simulink library "SUB_L4_Task_20ms"  (R2018a)
settings: Solver=VariableStepAuto  StartTime=0.0  StopTime=10.0  RelTol=1e-3
undefined symbols (not defined in the file or in its folder): DiscIntNeverNeededParam
settings Model: Creator=Chris.Balton  LastModifiedBy=Chris.Balton

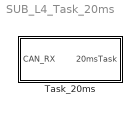
== system SUB_L4_Task_20ms ==
  Task_20ms : Subsystem  TreatAsAtomicUnit=on  SystemSampleTime=0.02

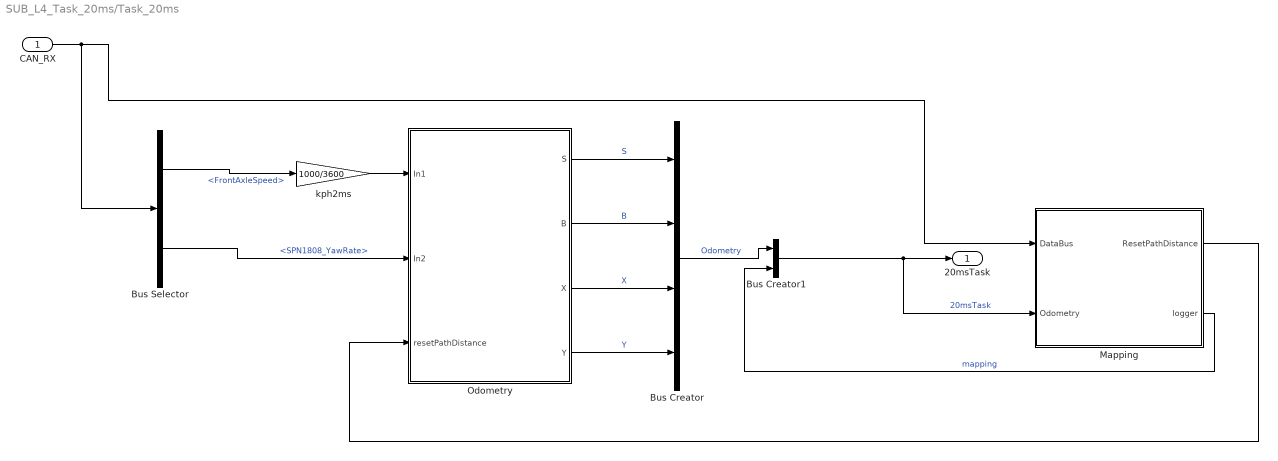
== system SUB_L4_Task_20ms/Task_20ms ==
  CAN_RX : Inport
  Bus Creator : BusCreator  Inputs=4
  Bus Creator1 : BusCreator  Inputs=2
  Bus Selector : BusSelector  OutputSignals=CAN.EBC2_0B.FrontAxleSpeed,CAN.VDC2_0B.SPN1808_YawRate
  Mapping : Subsystem
  Odometry : Subsystem
  kph2ms : Gain  Gain=1000/3600
  20msTask : Outport
  wires:
  Mapping/2(logger) -> Bus Creator1/2  "mapping"
  Mapping/1(ResetPathDistance) -> Odometry/3(resetPathDistance)
  Bus Creator1/1 -> Mapping/2(Odometry), 20msTask/1  "20msTask"
  Bus Creator/1 -> Bus Creator1/1  "Odometry"
  Odometry/4(Y) -> Bus Creator/4  "Y"
  Odometry/3(X) -> Bus Creator/3  "X"
  Odometry/2(B) -> Bus Creator/2  "B"
  Odometry/1(S) -> Bus Creator/1  "S"
  Bus Selector/2 -> Odometry/2(In2)  "<SPN1808_YawRate>"
  kph2ms/1 -> Odometry/1(In1)
  Bus Selector/1 -> kph2ms/1  "<FrontAxleSpeed>"
  CAN_RX/1 -> Mapping/1(DataBus), Bus Selector/1

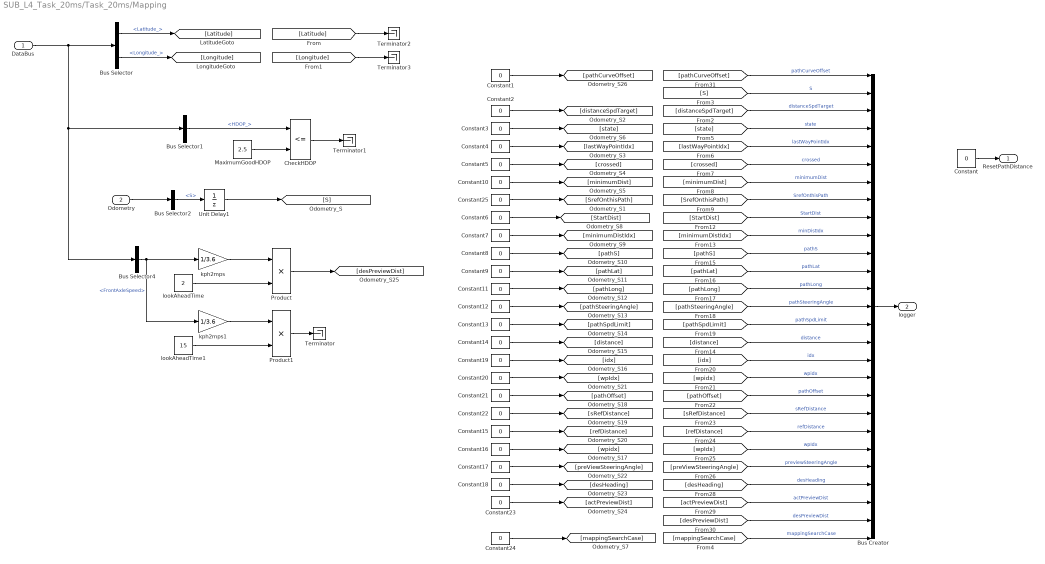
== system SUB_L4_Task_20ms/Task_20ms/Mapping ==
  DataBus : Inport
  Odometry : Inport  Port=2
  Bus Creator : BusCreator  Inputs=27
  Bus Selector : BusSelector  OutputSignals=CAN.PosRapidUpdate.Latitude_,CAN.PosRapidUpdate.Longitude_
  Bus Selector1 : BusSelector  OutputSignals=CAN.GNSSDOPs.HDOP_
  Bus Selector2 : BusSelector  OutputSignals=Odometry.S
  Bus Selector4 : BusSelector  OutputSignals=CAN.EBC2_0B.FrontAxleSpeed
  CheckHDOP : RelationalOperator  Operator=<=  OutDataTypeStr=boolean  RndMeth=Nearest
  Constant{,1..25} (26 alike) : Constant  Value=0
  MaximumGoodHDOP : Constant  Value=2.5
  Product : Product
  Product1 : Product
  Terminator{,1..3} (4 alike) : Terminator
  Unit Delay1 : UnitDelay  SampleTime=-1
  kph2mps : Gain  Gain=1/3.6
  kph2mps1 : Gain  Gain=1/3.6
  lookAheadTime : Constant  Value=2
  lookAheadTime1 : Constant  Value=15
  ResetPathDistance : Outport
  logger : Outport  Port=2
  wires:
  Constant25/1 -> [SrefOnthisPath]
  Constant24/1 -> [mappingSearchCase]
  Constant23/1 -> [actPreviewDist]
  Constant18/1 -> [desHeading]
  Constant17/1 -> [preViewSteeringAngle]
  Constant16/1 -> [wpidx]
  Constant19/1 -> [idx]
  Constant14/1 -> [distance]
  Constant13/1 -> [pathSpdLimit]
  Constant10/1 -> [minimumDist]
  Constant8/1 -> [pathS]
  Constant2/1 -> [distanceSpdTarget]
  Constant1/1 -> [pathCurveOffset]
  [mappingSearchCase] -> Bus Creator/27  "mappingSearchCase"
  [Longitude] -> Terminator3/1
  [Latitude] -> Terminator2/1
  kph2mps1/1 -> Product1/1
  Product1/1 -> Terminator/1
  lookAheadTime1/1 -> Product1/2
  Constant/1 -> ResetPathDistance/1
  [pathCurveOffset] -> Bus Creator/1  "pathCurveOffset"
  [desPreviewDist] -> Bus Creator/26  "desPreviewDist"
  [actPreviewDist] -> Bus Creator/25  "actPreviewDist"
  [desHeading] -> Bus Creator/24  "desHeading"
  Product/1 -> [desPreviewDist]
  lookAheadTime/1 -> Product/2
  kph2mps/1 -> Product/1
  Bus Selector4/1 -> kph2mps/1, kph2mps1/1  "<FrontAxleSpeed>"
  [preViewSteeringAngle] -> Bus Creator/23  "previewSteeringAngle"
  [wpIdx] -> Bus Creator/22  "wpIdx"
  [refDistance] -> Bus Creator/21  "refDistance"
  [sRefDistance] -> Bus Creator/20  "sRefDistance"
  [pathOffset] -> Bus Creator/19  "pathOffset"
  Constant20/1 -> [wpIdx]
  Constant15/1 -> [refDistance]
  Constant22/1 -> [sRefDistance]
  Constant21/1 -> [pathOffset]
  [wpidx] -> Bus Creator/18  "wpidx"
  [idx] -> Bus Creator/17  "idx"
  [distance] -> Bus Creator/16  "distance"
  Constant12/1 -> [pathSteeringAngle]
  Constant11/1 -> [pathLong]
  Constant9/1 -> [pathLat]
  [pathSpdLimit] -> Bus Creator/15  "pathSpdLimit"
  [pathSteeringAngle] -> Bus Creator/14  "pathSteeringAngle"
  [pathLong] -> Bus Creator/13  "pathLong"
  [pathLat] -> Bus Creator/12  "pathLat"
  [pathS] -> Bus Creator/11  "pathS"
  [minimumDistIdx] -> Bus Creator/10  "minDistIdx"
  Constant7/1 -> [minimumDistIdx]
  [StartDist] -> Bus Creator/9  "StartDist"
  Constant6/1 -> [StartDist]
  Bus Creator/1 -> logger/1
  [SrefOnthisPath] -> Bus Creator/8  "SrefOnthisPath"
  [minimumDist] -> Bus Creator/7  "minimumDist"
  [crossed] -> Bus Creator/6  "crossed"
  [lastWayPointIdx] -> Bus Creator/5  "lastWayPointIdx"
  [state] -> Bus Creator/4  "state"
  [distanceSpdTarget] -> Bus Creator/3  "distanceSpdTarget"
  [S] -> Bus Creator/2  "S"
  Constant5/1 -> [crossed]
  Constant4/1 -> [lastWayPointIdx]
  Unit Delay1/1 -> [S]
  DataBus/1 -> Bus Selector/1, Bus Selector1/1, Bus Selector4/1
  Constant3/1 -> [state]
  Bus Selector2/1 -> Unit Delay1/1  "<S>"
  Odometry/1 -> Bus Selector2/1
  CheckHDOP/1 -> Terminator1/1
  MaximumGoodHDOP/1 -> CheckHDOP/2
  Bus Selector1/1 -> CheckHDOP/1  "<HDOP_>"
  Bus Selector/1 -> [Latitude]  "<Latitude_>"
  Bus Selector/2 -> [Longitude]  "<Longitude_>"

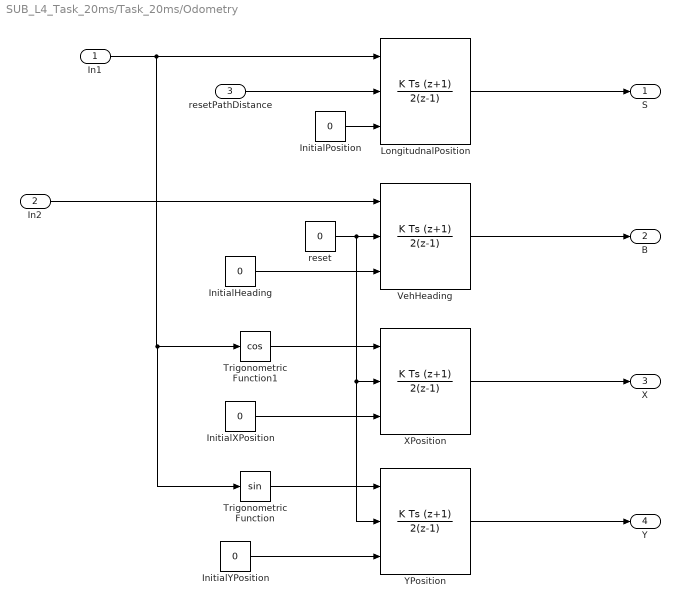
== system SUB_L4_Task_20ms/Task_20ms/Odometry ==
  In1 : Inport
  In2 : Inport  Port=2
  resetPathDistance : Inport  Port=3
  InitialHeading : Constant  Value=0
  InitialPosition : Constant  Value=0
  InitialXPosition : Constant  Value=0
  InitialYPosition : Constant  Value=0
  LongitudnalPosition : DiscreteIntegrator  IntegratorMethod=Integration: Trapezoidal  ExternalReset=rising  InitialConditionSource=external  SampleTime=-1  ICPrevOutput=DiscIntNeverNeededParam  ICPrevScaledInput=DiscIntNeverNeededParam
  Trigonometric Function : Trigonometry
  Trigonometric Function1 : Trigonometry  Operator=cos
  VehHeading : DiscreteIntegrator  IntegratorMethod=Integration: Trapezoidal  ExternalReset=rising  InitialConditionSource=external  SampleTime=-1  ICPrevOutput=DiscIntNeverNeededParam  ICPrevScaledInput=DiscIntNeverNeededParam
  XPosition : DiscreteIntegrator  IntegratorMethod=Integration: Trapezoidal  ExternalReset=rising  InitialConditionSource=external  SampleTime=-1  ICPrevOutput=DiscIntNeverNeededParam  ICPrevScaledInput=DiscIntNeverNeededParam
  YPosition : DiscreteIntegrator  IntegratorMethod=Integration: Trapezoidal  ExternalReset=rising  InitialConditionSource=external  SampleTime=-1  ICPrevOutput=DiscIntNeverNeededParam  ICPrevScaledInput=DiscIntNeverNeededParam
  reset : Constant  Value=0
  S : Outport
  B : Outport  Port=2
  X : Outport  Port=3
  Y : Outport  Port=4
  wires:
  reset/1 -> VehHeading/2, YPosition/2, XPosition/2
  InitialYPosition/1 -> YPosition/3
  XPosition/1 -> X/1
  LongitudnalPosition/1 -> S/1
  In1/1 -> LongitudnalPosition/1, Trigonometric Function1/1, Trigonometric Function/1
  YPosition/1 -> Y/1
  resetPathDistance/1 -> LongitudnalPosition/2
  Trigonometric Function/1 -> YPosition/1
  VehHeading/1 -> B/1
  Trigonometric Function1/1 -> XPosition/1
  In2/1 -> VehHeading/1
  InitialXPosition/1 -> XPosition/3
  InitialHeading/1 -> VehHeading/3
  InitialPosition/1 -> LongitudnalPosition/3
